simulink model "Sim5_OrthogonalArm_XY_OA"  (R2021b)
settings: Solver=VariableStepAuto  StartTime=0.0  StopTime=Inf  RelTol=1e-3
InitFcn:
  | Sim5_Status = 0;
  | set_param('Sim1_Supervisor_OA','SimulationCommand','update');
  | GUI = evalin('base','GUI_handle');
StopFcn:
  | Sim5_Status = 1;
  | set_param('Sim1_Supervisor_OA','SimulationCommand','update');
  | run('AutomoveData.m')
undefined symbols (not defined in the file or in its folder): ArmInitPos, armInitPos, BOXPos, dt, Twist
libraries: robotlib x5, realtime_pacer_lib x1
CloseFcn:
  | set(findobj(GUI,'Tag','open_sim5'),'Value','Close');
  | set(findobj(GUI,'Tag','open_sim5'),'Enable','on');
  | set(findobj(GUI,'Tag','start_sim5'),'Value','Stop');
  | set(findobj(GUI,'Tag','start_sim5'),'Enable','off');
settings Model: Creator=shdet  LastModifiedBy=Hibik
settings SolverCC: AlgebraicLoopSolver=TrustRegion
settings DebuggingCC: SFMachineParentedDataDiag=warning
settings SFSimCC: CustomCodeUndefinedFunction=UseInterfaceOnly

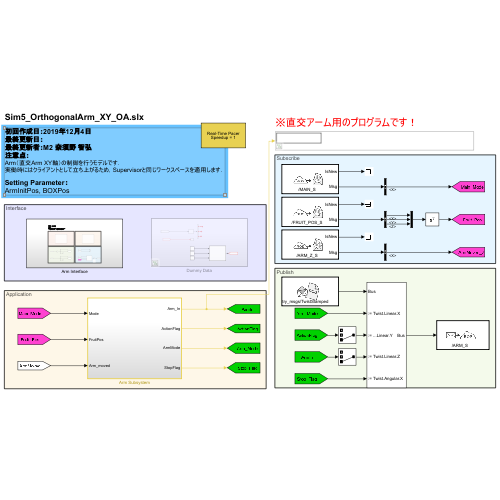
[thumbnail: Simulink's stored preview of the top-level diagram]
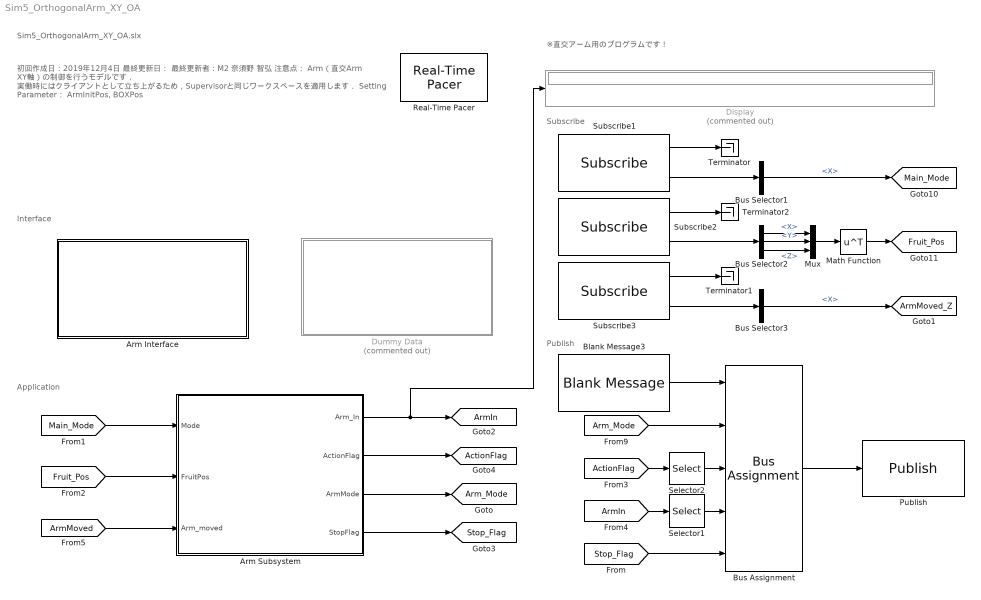
== system Sim5_OrthogonalArm_XY_OA ==
  note: Interface
  note: 初回作成日：2019年12月4日
      | 最終更新日：
      | 最終更新者：M2 奈須野 智弘
      | 注意点：
      | Arm（直交Arm XY軸）の制御を行うモデルです．
      | 実働時にはクライアントとして立ち上がるため，Supervisorと同じワークスペースを適用します．
      |
      | Setting Parameter：
      | ArmInitPos, BOXPos
  note: Application
  note: Publish
  note: Subscribe
  note: Sim5_OrthogonalArm_XY_OA.slx
  note: ※直交アーム用のプログラムです！
  Arm Interface : Subsystem
  Arm Subsystem : Subsystem  TreatAsAtomicUnit=on
  Blank Message3 : robotlib/Blank Message  messageClass=Message  entityType=geometry_msgs/TwistStamped  messageType=geometry_msgs/TwistStamped  SampleTime=inf  legacyBusStruct=off
  Bus Assignment : BusAssignment  AssignedSignals=Twist.Linear.X,Twist.Linear.Y,Twist.Linear.Z,Twist.Angular.X
  Bus Selector1 : BusSelector  OutputSignals=Twist.Linear.X
  Bus Selector2 : BusSelector  OutputSignals=Twist.Linear.X,Twist.Linear.Y,Twist.Linear.Z
  Bus Selector3 : BusSelector  OutputSignals=Twist.Linear.X
  Display : Display  Commented=on
  Dummy Data : Subsystem  Commented=on
  Math Function : Math  Operator=transpose  SignedPower=on  SaturateOnIntegerOverflow=on
  Mux : Mux  Inputs=3
  Publish : robotlib/Publish  topicSource=Specify your own  topic=/ARM_S  messageType=geometry_msgs/TwistStamped  legacyBusStruct=off  messageQueueLength=1
  Real-Time Pacer : realtime_pacer_lib/Real-Time Pacer  simTimePerRealTime=1
      settings: SourceProductName=Real-Time Pacer
  Selector1 : Selector  InputPortWidth=3  IndexOptions=Index vector (dialog)  Indices=3  OutputSizes=1
  Selector2 : Selector  InputPortWidth=3  IndexOptions=Index vector (dialog)  Indices=3  OutputSizes=1
  Subscribe1 : robotlib/Subscribe  topicSource=Specify your own  topic=/MAIN_S  messageType=geometry_msgs/TwistStamped  SampleTime=dt  legacyBusStruct=off  messageQueueLength=1
  Subscribe2 : robotlib/Subscribe  topicSource=Specify your own  topic=/FRUIT_POS_S  messageType=geometry_msgs/TwistStamped  SampleTime=dt  legacyBusStruct=off  messageQueueLength=1
  Subscribe3 : robotlib/Subscribe  topicSource=Specify your own  topic=/ARM_Z_S  messageType=geometry_msgs/TwistStamped  SampleTime=dt  legacyBusStruct=off  messageQueueLength=1
  Terminator : Terminator
  Terminator1 : Terminator
  Terminator2 : Terminator
  tag scope: ActionFlag=global, ArmIn=global, ArmMoved_Z=global, Arm_Mode=global, Fruit_Pos=global, Main_Mode=global, Stop_Flag=global
  wires:
  Subscribe1/2 -> Bus Selector1/1
  Bus Selector2/2 -> Mux/2  "<Y>"
  Arm Subsystem/3(ArmMode) -> [Arm_Mode]
  [Arm_Mode] -> Bus Assignment/2
  Subscribe2/1 -> Terminator2/1
  Math Function/1 -> [Fruit_Pos]
  Blank Message3/1 -> Bus Assignment/1
  Subscribe1/1 -> Terminator/1
  Arm Subsystem/2(ActionFlag) -> [ActionFlag]
  Bus Selector2/3 -> Mux/3  "<Z>"
  Bus Selector2/1 -> Mux/1  "<X>"
  [Main_Mode] -> Arm Subsystem/1(Mode)
  Mux/1 -> Math Function/1
  [Fruit_Pos] -> Arm Subsystem/2(FruitPos)
  Bus Assignment/1 -> Publish/1
  [ArmMoved] -> Arm Subsystem/3(Arm_moved)
  Arm Subsystem/1(Arm_In) -> Display/1, [ArmIn]
  Subscribe2/2 -> Bus Selector2/1
  Bus Selector1/1 -> [Main_Mode]  "<X>"
  Bus Selector3/1 -> [ArmMoved_Z]  "<X>"
  Subscribe3/1 -> Terminator1/1
  Subscribe3/2 -> Bus Selector3/1
  [ActionFlag] -> Selector2/1
  Selector2/1 -> Bus Assignment/3
  [ArmIn] -> Selector1/1
  Selector1/1 -> Bus Assignment/4
  Arm Subsystem/4(StopFlag) -> [Stop_Flag]
  [Stop_Flag] -> Bus Assignment/5

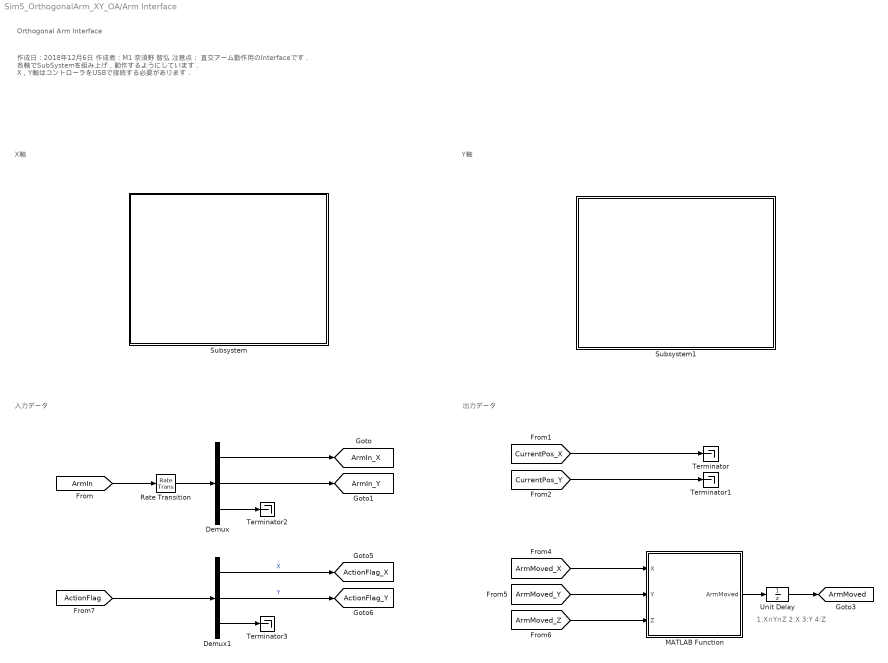
== system Sim5_OrthogonalArm_XY_OA/Arm Interface ==
  note: 出力データ
  note: 1:X∩Y∩Z
      | 2:X
      | 3:Y
      | 4:Z
  note: Orthogonal Arm Interface
  note: 作成日：2018年12月6日
      | 作成者：M1 奈須野 智弘
      | 注意点：
      | 直交アーム動作用のInterfaceです．
      | 各軸でSubSystemを組み上げ，動作するようにしています．
      | X，Y軸はコントローラをUSBで接続する必要があります．
  note: X軸
  note: 入力データ
  note: Y軸
  Demux : Demux  Outputs=3
  Demux1 : Demux  Outputs=3
  MATLAB Function : MATLAB Function  TreatAsAtomicUnit=on
  Rate Transition : RateTransition  OutPortSampleTime=0.1
  Subsystem : Subsystem
  Subsystem1 : Subsystem
  Terminator{,1..3} (4 alike) : Terminator
  Unit Delay : UnitDelay  SampleTime=-1  HasFrameUpgradeWarning=on
  tag scope: ActionFlag_X=global, ActionFlag_Y=global, ArmIn_X=global, ArmIn_Y=global, ArmMoved=global
  wires:
  [ArmMoved_Z] -> MATLAB Function/3(Z)
  MATLAB Function/1(ArmMoved) -> Unit Delay/1
  Rate Transition/1 -> Demux/1
  Demux/2 -> [ArmIn_Y]
  Demux1/2 -> [ActionFlag_Y]  "Y"
  Demux1/1 -> [ActionFlag_X]  "X"
  [ActionFlag] -> Demux1/1
  [ArmMoved_Y] -> MATLAB Function/2(Y)
  [CurrentPos_X] -> Terminator/1
  [ArmIn] -> Rate Transition/1
  Demux/1 -> [ArmIn_X]
  [CurrentPos_Y] -> Terminator1/1
  Unit Delay/1 -> [ArmMoved]
  [ArmMoved_X] -> MATLAB Function/1(X)
  Demux/3 -> Terminator2/1
  Demux1/3 -> Terminator3/1

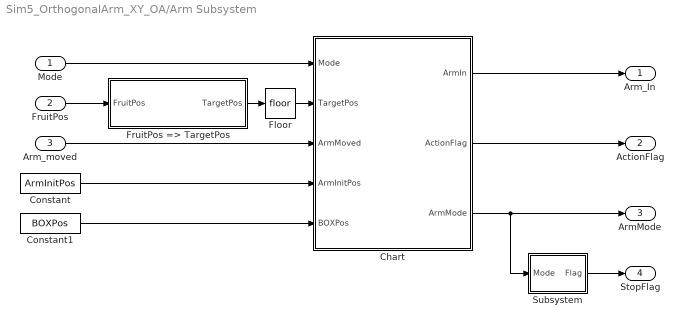
== system Sim5_OrthogonalArm_XY_OA/Arm Subsystem ==
  Mode : Inport  PortDimensions=1
  FruitPos : Inport  Port=2
  Arm_moved : Inport  Port=3
  Chart : Stateflow chart  TreatAsAtomicUnit=on
  Constant : Constant  Value=ArmInitPos  VectorParams1D=off
  Constant1 : Constant  Value=BOXPos  VectorParams1D=off
  Floor : Rounding
  FruitPos => TargetPos : MATLAB Function  TreatAsAtomicUnit=on
  Subsystem : Subsystem
  Arm_In : Outport  InitialOutput=armInitPos  VectorParamsAs1DForOutWhenUnconnected=off
  ActionFlag : Outport  Port=2  VectorParamsAs1DForOutWhenUnconnected=off
  ArmMode : Outport  Port=3  PortDimensions=1  InitialOutput=0  VectorParamsAs1DForOutWhenUnconnected=off
  StopFlag : Outport  Port=4  PortDimensions=1  InitialOutput=0  VectorParamsAs1DForOutWhenUnconnected=off
  wires:
  Chart/1(ArmIn) -> Arm_In/1
  Mode/1 -> Chart/1(Mode)
  FruitPos/1 -> FruitPos => TargetPos/1(FruitPos)
  Arm_moved/1 -> Chart/3(ArmMoved)
  Chart/2(ActionFlag) -> ActionFlag/1
  Constant/1 -> Chart/4(ArmInitPos)
  FruitPos => TargetPos/1(TargetPos) -> Floor/1
  Constant1/1 -> Chart/5(BOXPos)
  Floor/1 -> Chart/2(TargetPos)
  Chart/3(ArmMode) -> Subsystem/1(Mode), ArmMode/1
  Subsystem/1(Flag) -> StopFlag/1

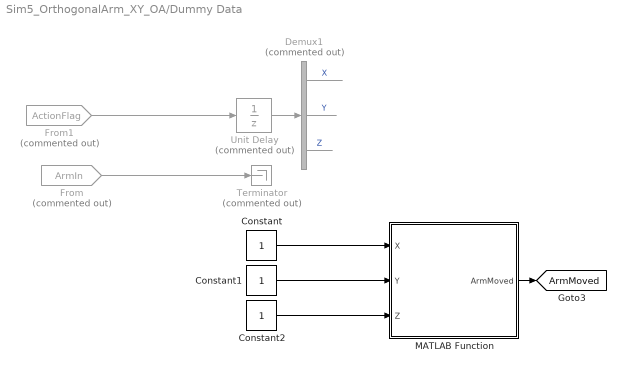
== system Sim5_OrthogonalArm_XY_OA/Dummy Data ==
  Constant : Constant
  Constant1 : Constant
  Constant2 : Constant
  Demux1 : Demux  Commented=on  Outputs=3
  From : From  Commented=on  GotoTag=ArmIn  TagVisibility=global
  From1 : From  Commented=on  GotoTag=ActionFlag  TagVisibility=global
  MATLAB Function : MATLAB Function  TreatAsAtomicUnit=on
  Terminator : Terminator  Commented=on
  Unit Delay : UnitDelay  Commented=on  SampleTime=-1  HasFrameUpgradeWarning=on
  tag scope: ArmMoved=global
  wires:
  From/1 -> Terminator/1
  Unit Delay/1 -> Demux1/1
  Demux1/1 -> ?  "X"
  Demux1/2 -> ?  "Y"
  Demux1/3 -> ?  "Z"
  MATLAB Function/1(ArmMoved) -> [ArmMoved]
  From1/1 -> Unit Delay/1
  Constant/1 -> MATLAB Function/1(X)
  Constant1/1 -> MATLAB Function/2(Y)
  Constant2/1 -> MATLAB Function/3(Z)

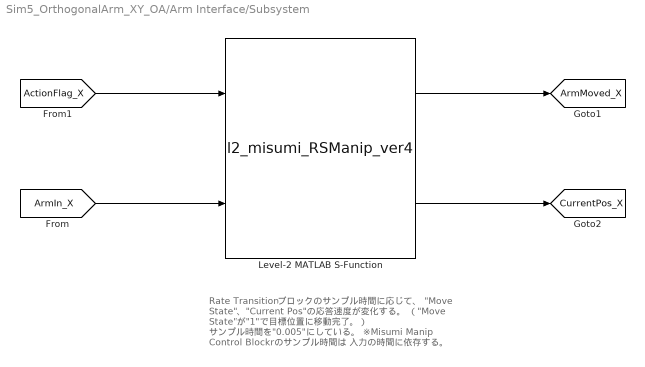
== system Sim5_OrthogonalArm_XY_OA/Arm Interface/Subsystem ==
  note: Rate Transitionブロックのサンプル時間に応じて、
      | "Move State"、"Current Pos"の応答速度が変化する。
      | （"Move State"が"1"で目標位置に移動完了。）
      | サンプル時間を"0.005"にしている。
      |
      | ※Misumi Manip Control Blocknのサンプル時間は
      | 入力の時間に依存する。
  Level-2 MATLAB S-Function : M-S-Function  FunctionName=l2_misumi_RSManip_ver4  Parameters=comport, initPos, speed  mask{comport='COM9', initPos=ArmInitPos(1), speed=100}
      mask prompts: comport "Port Number"; initPos "Init Position"
      mask help:
      | MisumiRS Manip Control Block ver1.
      | Rang of Init and Target Pos is 0 to 200 for RS306 (y-axis).
      mask Display:
      | disp('MisumiRS Manip Control Block');
      | port_label('input',1,'Act.Flag');
      | port_label('input',2,'Target Pos');
      | port_label('output',1,'Moved State');
      | port_label('output',2,'Current Pos');
  tag scope: ArmMoved_X=global, CurrentPos_X=global
  wires:
  [ActionFlag_X] -> Level-2 MATLAB S-Function/1
  Level-2 MATLAB S-Function/1 -> [ArmMoved_X]
  Level-2 MATLAB S-Function/2 -> [CurrentPos_X]
  [ArmIn_X] -> Level-2 MATLAB S-Function/2

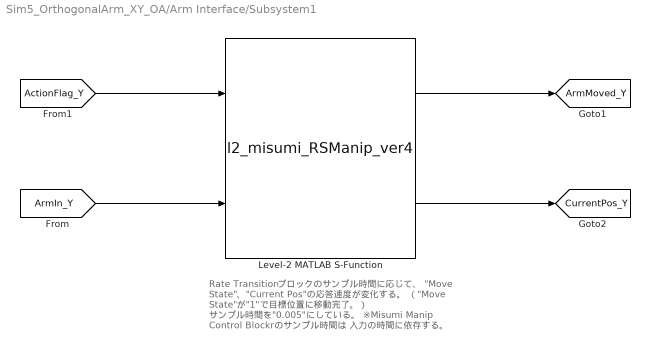
== system Sim5_OrthogonalArm_XY_OA/Arm Interface/Subsystem1 ==
  note: Rate Transitionブロックのサンプル時間に応じて、
      | "Move State"、"Current Pos"の応答速度が変化する。
      | （"Move State"が"1"で目標位置に移動完了。）
      | サンプル時間を"0.005"にしている。
      |
      | ※Misumi Manip Control Blocknのサンプル時間は
      | 入力の時間に依存する。
  Level-2 MATLAB S-Function : M-S-Function  FunctionName=l2_misumi_RSManip_ver4  Parameters=comport, initPos, speed  mask{comport='COM8', initPos=ArmInitPos(2), speed=100}
      mask prompts: comport "Port Number"; initPos "Init Position"
      mask help:
      | MisumiRS Manip Control Block ver1.
      | Rang of Init and Target Pos is 0 to 200 for RS306 (y-axis).
      mask Display:
      | disp('MisumiRS Manip Control Block');
      | port_label('input',1,'Act.Flag');
      | port_label('input',2,'Target Pos');
      | port_label('output',1,'Moved State');
      | port_label('output',2,'Current Pos');
  tag scope: ArmMoved_Y=global, CurrentPos_Y=global
  wires:
  [ActionFlag_Y] -> Level-2 MATLAB S-Function/1
  Level-2 MATLAB S-Function/2 -> [CurrentPos_Y]
  Level-2 MATLAB S-Function/1 -> [ArmMoved_Y]
  [ArmIn_Y] -> Level-2 MATLAB S-Function/2

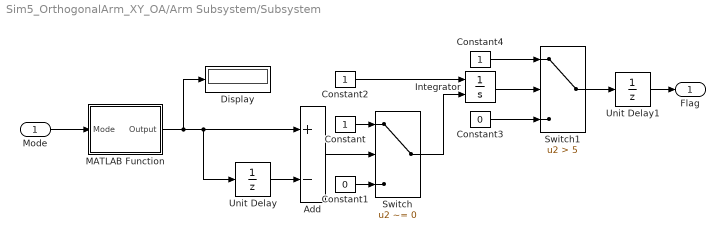
== system Sim5_OrthogonalArm_XY_OA/Arm Subsystem/Subsystem ==
  Mode : Inport
  Add : Sum  Inputs=+-
  Constant : Constant
  Constant1 : Constant  Value=0
  Constant2 : Constant
  Constant3 : Constant  Value=0
  Constant4 : Constant
  Display : Display
  Integrator : Integrator  ExternalReset=level
  MATLAB Function : MATLAB Function  TreatAsAtomicUnit=on
  Switch : Switch  Criteria=u2 ~= 0
  Switch1 : Switch  Criteria=u2 > Threshold  Threshold=5
  Unit Delay : UnitDelay  SampleTime=-1  HasFrameUpgradeWarning=on
  Unit Delay1 : UnitDelay  SampleTime=-1  HasFrameUpgradeWarning=on
  Flag : Outport  VectorParamsAs1DForOutWhenUnconnected=off
  wires:
  Unit Delay/1 -> Add/2
  Add/1 -> Switch/2
  Constant/1 -> Switch/1
  Constant1/1 -> Switch/3
  Constant2/1 -> Integrator/1
  Switch/1 -> Integrator/2
  Switch1/1 -> Unit Delay1/1
  Integrator/1 -> Switch1/2
  Constant3/1 -> Switch1/3
  Constant4/1 -> Switch1/1
  Mode/1 -> MATLAB Function/1(Mode)
  MATLAB Function/1(Output) -> Unit Delay/1, Add/1, Display/1
  Unit Delay1/1 -> Flag/1

== matlab function Sim5_OrthogonalArm_XY_OA/Arm Interface/MATLAB Function ==
  data: X input; ArmMoved output; Y input; Z input
function ArmMoved = fcn(X,Y,Z)



if X == 1 && Y == 1 && Z == 1
    ArmMoved_XYZ = 1;
else
    ArmMoved_XYZ = 0;
end

ArmMoved = [ArmMoved_XYZ, X, Y, Z];

== matlab function Sim5_OrthogonalArm_XY_OA/Arm Subsystem/FruitPos => TargetPos ==
  data: FruitPos input; TargetPos output
function TargetPos = fcn(FruitPos)

TargetPos = FruitPos;

if FruitPos(1) > 200
    TargetPos(1) = 0;
elseif FruitPos(1) < 0
    TargetPos(1) = 200;
else
    TargetPos(1) = 200 - FruitPos(1);
end
if FruitPos(2) > 200
    TargetPos(2) = 200;
elseif FruitPos(2) < 0
    TargetPos(2) = 0;
end
if FruitPos(3) > 470
    TargetPos(3) = 470;
elseif FruitPos(3) < 60
    TargetPos(3) = 60;
end

== matlab function Sim5_OrthogonalArm_XY_OA/Dummy Data/MATLAB Function ==
  data: X input; ArmMoved output; Y input; Z input
function ArmMoved = fcn(X,Y,Z)



if X == 1 && Y == 1 && Z == 1
    ArmMoved_XYZ = 1;
else
    ArmMoved_XYZ = 0;
end

ArmMoved = [ArmMoved_XYZ, X, Y, Z];

== matlab function Sim5_OrthogonalArm_XY_OA/Arm Subsystem/Subsystem/MATLAB Function ==
  data: Mode input; Output output
function Output = fcn(Mode)

if Mode == 1 || Mode == 4 || Mode == 11 || Mode == 12 || Mode == 21 || Mode == 22 ...
        || Mode == 41 || Mode == 42
    Output = Mode;
else
    Output = randi(100);
end

== stateflow chart Sim5_OrthogonalArm_XY_OA/Arm Subsystem/Chart ==
  state Mode0_Z2/
    % Move Init. Pos. Z
    entry:
    ActionFlag = [0, 0, 1];
    ArmIn = ArmInitPos;
  state Wait01/
    % Wait for input
    entry:
    ArmMode = 100;
    ActionFlag = [0,0,0];
  state Arm_Move/
    state Return_InitPositionX/
      % x座標アームを原点移動
      entry:
      ArmMode = 21;
      state Mode0_X/
        % Move Init. Pos. X
        entry:
        ArmMode = 21;
        ActionFlag = [1,0,0];
        ArmIn = ArmInitPos;
      state Finished_X/
        entry:
        ArmMode = 22;
        ActionFlag = [0,0,0];
      (default) -> Arm_Move.Return_InitPositionX.Mode0_X
      Arm_Move.Return_InitPositionX.Mode0_X -> Arm_Move.Return_InitPositionX.Finished_X : after(0.5,sec)[ArmMoved(2) == 1]
    state Arm_MoveTarget1/
      %TargetPosの座標にアーム移動
      entry:
      ArmMode = 1;
      NeedTime = abs(ArmInitPos(3)-TargetPos(3))/100;
      state Mode1/
        % Move Y
        entry:
        ArmMode = 1;
        ActionFlag = [0,1,0];
        ArmIn = TargetPos;
      state Mode2/
        % Move Z
        entry:
        ArmMode = 2;
        ActionFlag = [0,0,1];
        ArmIn = TargetPos;
      state Finished_Z/
        entry:ArmMode = 3;
        ActionFlag = [0,0,0];
      state Mode3/
        % Move X
        entry:
        ArmMode = 4;
        ActionFlag = [1,0,0];
        ArmIn = TargetPos;
      (default) -> Mode1
      Mode1 -> Mode2 : after(0.5,sec)[ArmMoved(3) == 1]
      Mode2 -> Finished_Z : after(5,sec)
      Finished_Z -> Mode3 : [Mode == 42]
    state Return_InitPositionZY/
      % z,y座標アームを原点移動
      entry:
      ArmMode = 31;
      NeedTime = abs(ArmInitPos(3)-TargetPos(3))/100;
      state Mode0_Z/
        % Move Init. Pos. Z
        entry:
        ArmMode = 31;
        ActionFlag = [0,0,1];
        ArmIn = ArmInitPos;
      state Mode0_Y/
        % Move Init. Pos. Y
        entry:
        ArmMode = 32;
        ActionFlag = [0,1,0]
        ArmIn = ArmInitPos;
      state Finished_X/
        entry:
        ArmMode = 33;
        ActionFlag = [0,0,0];
      (default) -> Arm_Move.Return_InitPositionZY.Mode0_Z
      Arm_Move.Return_InitPositionZY.Mode0_Z -> Arm_Move.Return_InitPositionZY.Mode0_Y : after(5,sec)
      Arm_Move.Return_InitPositionZY.Mode0_Y -> Arm_Move.Return_InitPositionZY.Finished_X : after(2,sec)[ArmMoved(3) == 1]
    state Wait5/
      % Wait
      entry:
      ArmMode = 10;
      ActionFlag = [0,0,0];
    (default) -> Arm_MoveTarget1
    Wait5 -> Return_InitPositionX : [Mode == 51 || Mode == 47]
    Return_InitPositionX -> Return_InitPositionZY : [Mode == 62 || Mode == 52]
    Mode3 -> Wait5 : after(0.5,sec)[ArmMoved(2) == 1]
  state Return_InitPosition2/
    % ArmInitPosの座標にアームを移動（未終了時）
    entry:
    ArmMode = 41;
    state Mode0_X/
      % Move Init. Pos. X
      entry:
      ArmMode = 41;
      ActionFlag = [1,0,0];
      ArmIn = ArmInitPos;
    state Mode0_Y/
      % Move Init. Pos. Y
      entry:
      ArmMode = 42;
      ActionFlag = [0,1,0];
      ArmIn = ArmInitPos;
    state Mode0_Z/
      % Move Init. Pos. Z
      entry:
      ArmMode = 43;
      ActionFlag = [0,0,1];
      ArmIn = ArmInitPos;
    (default) -> Return_InitPosition2.Mode0_X
    Return_InitPosition2.Mode0_X -> Return_InitPosition2.Mode0_Y : after(0.5,sec)[ArmMoved(2) == 1]
    Return_InitPosition2.Mode0_Y -> Return_InitPosition2.Mode0_Z : after(0.5,sec)[ArmMoved(3) == 1]
  (default) -> Mode0_Z2
  Mode0_Z2 -> Wait01 : after(5.0,sec)
  (junction 221) -> Wait01
  Wait01 -> Arm_Move : [Mode == 41]
  Return_InitPosition2.Mode0_Z -> (junction 221) : after(3.0,sec)
  Arm_Move -> Return_InitPosition2 : [Mode == 70]
  data: Mode input; TargetPos input; ArmIn output; ActionFlag output; ArmMode output; ArmMoved input; ArmInitPos input; BOXPos input; NeedTime local
